simulink model "main_smc"  (R2021b)
settings: Solver=ode45  StartTime=0.0  StopTime=80  FixedStep=0.1  RelTol=1e-4
libraries: slpidlib x6
(part 2 of 2)

== matlab function main_smc/u1 whit /u1 ==
  data: dz input; phi input; u1 output; theta input; dzd input; ddzd input; ms input; g input; wz input; epsilonz input; s_z input; u1_dis output
function [u1,u1_dis] = u1_function(dz,phi,theta,dzd,ddzd,ms,g,wz,epsilonz,s_z)

u1_dis = ms/(cos(theta)*cos(phi))*(epsilonz*tanh(s_z));
u1 = ms/(cos(theta)*cos(phi))*(wz*(dzd - dz) + ddzd + g) + ms/(cos(theta)*cos(phi))*(epsilonz*tanh(s_z));
end

== matlab function main_smc/u1 whit /u1 sign ==
  data: z_t input; z_t_1 input; u1_sign output; u1_dis input; u1_dis_t_1 input
function u1_sign  = u1_sing(z_t,z_t_1,u1_dis,u1_dis_t_1)
if (u1_dis-u1_dis_t_1) == 0
    u1_sign=0;
else
    u1_sign=sign( (z_t-z_t_1)/(u1_dis-u1_dis_t_1) );
end
end
